simulink model "simumod"  (R2021b)
settings: Solver=VariableStepAuto  StartTime=0.0  StopTime=1e-4  RelTol=1e-3
model workspace (MAT data in the model file):
  sinput = Simulink.Parameter
  sinput.DataType = 'auto'
  sinput.Complexity = 'real'
  sinput.Dimensions = [0 0]
settings Model: Creator=Phecda  LastModifiedBy=Phecda

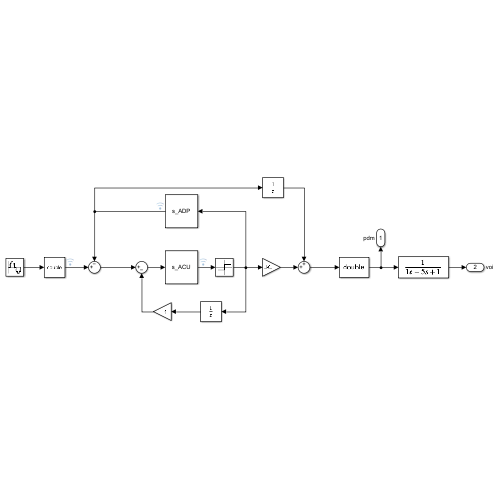
[thumbnail: Simulink's stored preview of the top-level diagram]
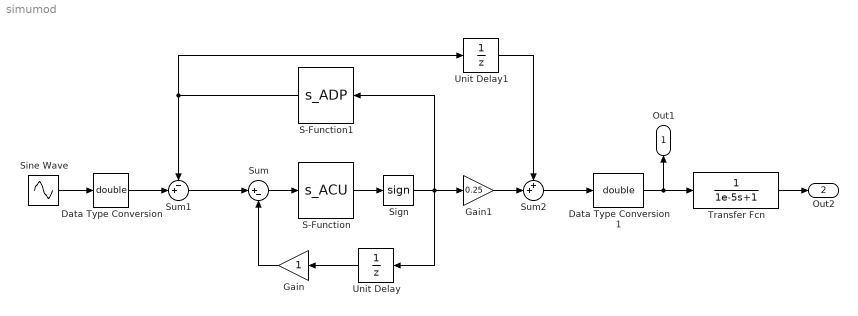
== system simumod ==
  Data Type Conversion : DataTypeConversion  OutDataTypeStr=double  RndMeth=Round
  Data Type Conversion1 : DataTypeConversion  OutMin=[0]  OutMax=[1]  OutDataTypeStr=double  RndMeth=Round
  Gain : Gain
  Gain1 : Gain  Gain=0.25
  S-Function : S-Function  FunctionName=s_ACU  Parameters=fs,k  SFunctionDeploymentMode=off  EnableBusSupport=off  mask{fs=50e6, k=1}
  S-Function1 : S-Function  FunctionName=s_ADP  Parameters=fs,b,q  SFunctionDeploymentMode=off  EnableBusSupport=off  mask{fs=50e6, b=0.25, q=0.5}
  Sign : Signum
  Sine Wave : Sin  Amplitude=0.5  Frequency=1e5  Samples=1000000  SampleTime=0.02e-6
  Sum : Sum  Inputs=|+-
  Sum1 : Sum  Inputs=-+|  RndMeth=Round
  Sum2 : Sum  Inputs=++|  RndMeth=Round
  Transfer Fcn : TransferFcn  Denominator=[1e-5 1]
  Unit Delay : UnitDelay  SampleTime=0.02e-6  HasFrameUpgradeWarning=on
  Unit Delay1 : UnitDelay  SampleTime=0.02e-6  HasFrameUpgradeWarning=on
  Out1 : Outport  SignalName=pdm
  Out2 : Outport  Port=2  SignalName=voi
  wires:
  Sine Wave/1 -> Data Type Conversion/1
  Transfer Fcn/1 -> Out2/1
  Data Type Conversion1/1 -> Transfer Fcn/1, Out1/1
  Sum/1 -> S-Function/1
  S-Function/1 -> Sign/1
  Sign/1 -> Gain1/1, S-Function1/1, Unit Delay/1
  Unit Delay/1 -> Gain/1
  Gain/1 -> Sum/2
  Data Type Conversion/1 -> Sum1/2
  S-Function1/1 -> Unit Delay1/1, Sum1/1
  Sum1/1 -> Sum/1
  Sum2/1 -> Data Type Conversion1/1
  Unit Delay1/1 -> Sum2/1
  Gain1/1 -> Sum2/2
